simulink model "AperiodicSISOControl"  (R2025b)
settings: Solver=FixedStepAuto  StartTime=0.0  StopTime=50  FixedStep=0.01  RelTol=1e-3  EnableMultiTasking=on
libraries: AVE_Library x1
settings Model: Creator=Scythe  LastModifiedBy=damerius
settings SolverCC: ConcurrentTasks=on
settings DataIOCC: SaveOutput=off  SignalLogging=off  DSMLogging=off  SaveTime=off  ReturnWorkspaceOutputs=off
settings OptimizationCC: DefaultParameterBehavior=Inlined  EnhancedBackFolding=on  PassReuseOutputArgsAs=Individual arguments  ZeroExternalMemoryAtStartup=off  ZeroInternalMemoryAtStartup=off  SimCompilerOptimization=on  OptimizeBlockOrder=speed  DifferentSizesBufferReuse=on  OptimizationCustomize=off  EfficientTunableParamExpr=on
settings DebuggingCC: ParameterTunabilityLossMsg=error  UnconnectedInputMsg=warning  UnconnectedOutputMsg=warning  UnconnectedLineMsg=warning
settings HardwareCC: ProdBitPerLong=64.0  ProdHWDeviceType=Intel->x86-64 (Linux 64)  TargetBitPerLong=64.0  TargetBitPerPointer=64.0  TargetBitPerSizeT=64.0  TargetBitPerPtrDiffT=64.0  TargetLargestAtomicFloat=Float  TargetIntDivRoundTo=Zero  TargetEndianess=LittleEndian  TargetWordSize=64.0  TargetHWDeviceType=Intel->x86-64 (Linux 64)  ProdEqTarget=off
settings ModelReferenceCC: EnableRefExpFcnMdlSchedulingChecks=on
settings SFSimCC: SimGenImportedTypeDefs=on  SimTargetLang=C++  SimDLTargetLibrary=mkl-dnn
settings RTWCC: SystemTargetFile=ert.tlc  GenCodeOnly=on  PackageGeneratedCodeAndArtifacts=on  PackageName=PackNGo  TemplateMakefile=ert_default_tmf  Toolchain=CMake  DataTypeReplacement=CDataTypesFixedWidth  TargetLang=C++  Description=Embedded Coder
settings CodeAppCC: ForceParamTrailComments=on  IgnoreCustomStorageClasses=off  MaxIdLength=128.0  OperatorAnnotations=on  SimulinkDataObjDesc=on  SFDataObjDesc=on  InsertBlockDesc=on  StateflowObjectComments=on  MATLABSourceComments=on  UseSimReservedNames=on
settings ERTTargetCC: TargetOS=NativeThreadsExample  RootIOFormat=Structure reference  ERTCustomFileTemplate=example_file_process.tlc  IndentSize=4  NewlineStyle=LF  MaxLineWidth=256.0  MaxIdInt64=INT64_MAX  MinIdInt64=INT64_MIN  MaxIdUint64=UINT64_MAX  MaxIdInt32=INT32_MAX  MinIdInt32=INT32_MIN  MaxIdUint32=UINT32_MAX  MaxIdInt16=INT16_MAX  MinIdInt16=INT16_MIN  MaxIdUint16=UINT16_MAX  MaxIdInt8=INT8_MAX  MinIdInt8=INT8_MIN  MaxIdUint8=UINT8_MAX  DynamicArrayContainerType=coder::array  TargetLangStandard=C++20 (ISO)  CodeInterfacePackaging=C++ class  SubcomponentCodeInterfacePackaging=C++ class  SupportContinuousTime=on  SupportVariableSizeSignals=on

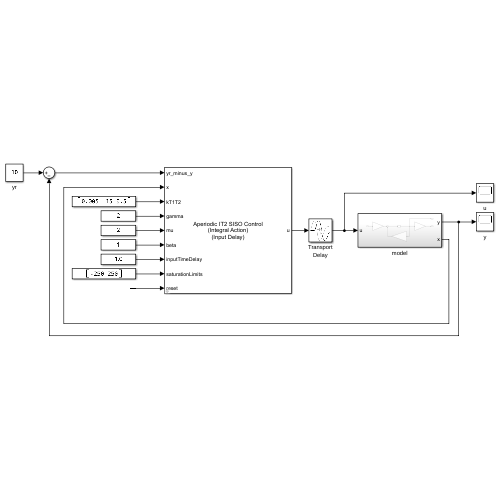
[thumbnail: Simulink's stored preview of the top-level diagram]
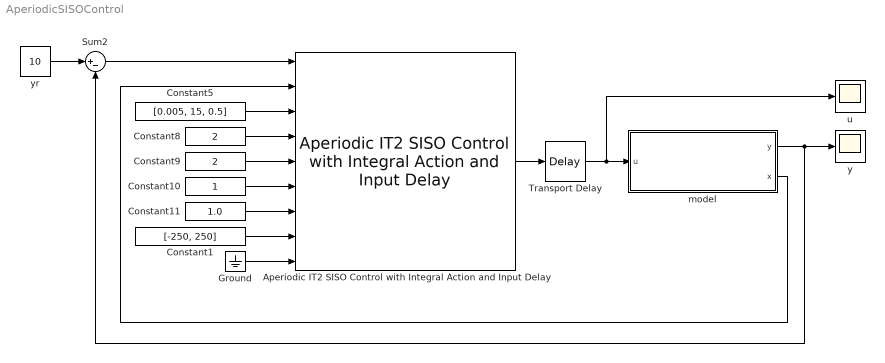
== system AperiodicSISOControl ==
  Aperiodic IT2 SISO Control with Integral Action and Input Delay : AVE_Library/Control/Aperiodic IT2 SISO Control with Integral Action and Input Delay  maxNumDelays=100  SampleTime=0.01
      settings: SourceProductName=AVE - Autonomous Vehicle Control Toolbox
  Constant1 : Constant  Value=[-250, 250]
  Constant10 : Constant
  Constant11 : Constant  Value=1.0
  Constant5 : Constant  Value=[0.005, 15, 0.5]
  Constant8 : Constant  Value=2
  Constant9 : Constant  Value=2
  Ground : Ground
  Sum2 : Sum  Inputs=|+-
  Transport Delay : TransportDelay  DelayTime=1.0
  model : Subsystem
  u : Scope
      settings: ActiveDisplayYMinimum=-312.5  ActiveDisplayYMaximum=312.5
  y : Scope
      settings: ActiveDisplayYMinimum=-1.2428015349797938  ActiveDisplayYMaximum=11.185213814818146  DataLoggingVariableName=ScopeData2
  yr : Constant  Value=10
  wires:
  Ground/1 -> Aperiodic IT2 SISO Control with Integral Action and Input Delay/9
  Constant1/1 -> Aperiodic IT2 SISO Control with Integral Action and Input Delay/8
  Constant11/1 -> Aperiodic IT2 SISO Control with Integral Action and Input Delay/7
  Constant10/1 -> Aperiodic IT2 SISO Control with Integral Action and Input Delay/6
  Constant9/1 -> Aperiodic IT2 SISO Control with Integral Action and Input Delay/5
  Constant8/1 -> Aperiodic IT2 SISO Control with Integral Action and Input Delay/4
  Constant5/1 -> Aperiodic IT2 SISO Control with Integral Action and Input Delay/3
  Transport Delay/1 -> u/1, model/1(u)
  model/2(x) -> Aperiodic IT2 SISO Control with Integral Action and Input Delay/2
  yr/1 -> Sum2/1
  model/1(y) -> y/1, Sum2/2
  Sum2/1 -> Aperiodic IT2 SISO Control with Integral Action and Input Delay/1
  Aperiodic IT2 SISO Control with Integral Action and Input Delay/1 -> Transport Delay/1

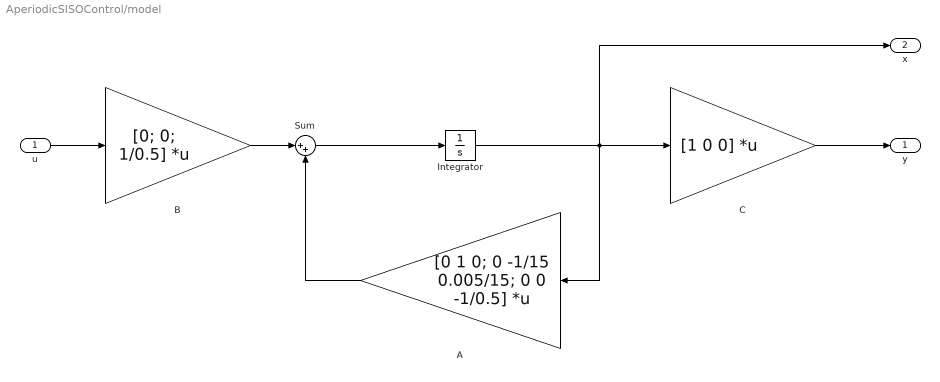
== system AperiodicSISOControl/model ==
  u : Inport
  A : Gain  Gain=[0 1 0; 0 -1/15 0.005/15; 0 0 -1/0.5]  Multiplication=Matrix(K*u)
  B : Gain  Gain=[0; 0; 1/0.5]  Multiplication=Matrix(K*u)
  C : Gain  Gain=[1 0 0]  Multiplication=Matrix(K*u)
  Integrator : Integrator
  Sum : Sum  Inputs=|++
  y : Outport
  x : Outport  Port=2
  wires:
  u/1 -> B/1
  B/1 -> Sum/1
  Sum/1 -> Integrator/1
  A/1 -> Sum/2
  Integrator/1 -> x/1, C/1, A/1
  C/1 -> y/1
